simulink model "valida_angulo"  (R2023a)
settings: Solver=VariableStepAuto  StartTime=0.0  StopTime=10  RelTol=1e-3
values from neighbouring files (symbols this model uses):
  B = 0.3441    [datos_planta.m]
  J = 0.0112    [datos_planta.m]
  Jv = 13576.379e-12    (= 1.3576379e-08)    [datos_planta.m]
  Ka = 0.2335    [datos_planta.m]
  Km = 0.147    [datos_planta.m]
  L = 0.52    [datos_planta.m]
  R = 1.6    [datos_planta.m]
  Tm = 0.41    [datos_planta.m]
settings Model: Creator=hiago.sodre  LastModifiedBy=hiago.sodre

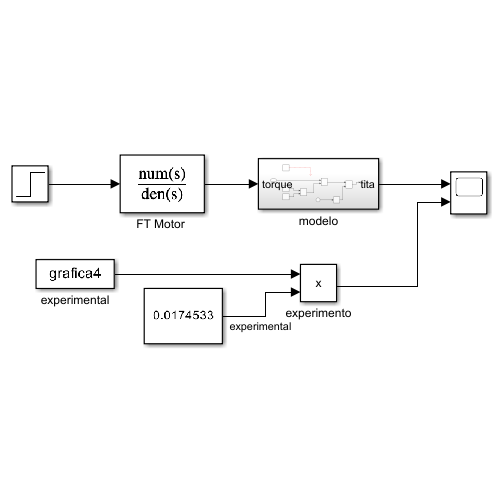
[thumbnail: Simulink's stored preview of the top-level diagram]
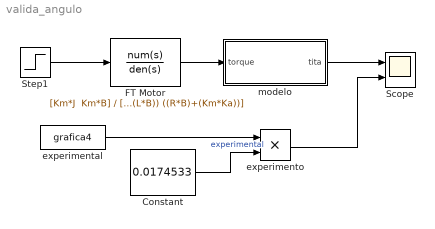
== system valida_angulo ==
  Constant : Constant  Value=0.0174533
  "FT Motor " : TransferFcn  Numerator="[Km*J  Km*B]"  Denominator=[L*J ((R*J)+(L*B)) ((R*B)+(Km*Ka))]
  Scope : Scope  NumInputPorts=2
  Step1 : Step  Time=0  After=5  SampleTime=0
  experimental : FromWorkspace  VariableName=grafica4
  experimento : Product  Inputs=**
  modelo : Subsystem
  wires:
  experimental/1 -> experimento/1
  Constant/1 -> experimento/2  "experimental"
  "FT Motor "/1 -> modelo/1(torque)
  Step1/1 -> "FT Motor "/1
  modelo/1(tita) -> Scope/1
  experimento/1 -> Scope/2

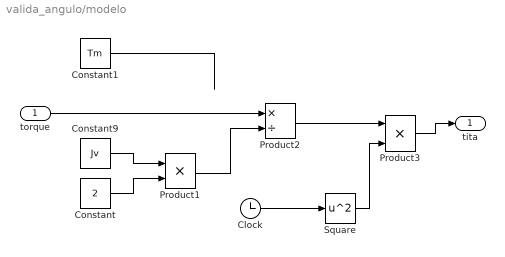
== system valida_angulo/modelo ==
  torque : Inport
  Clock : Clock
  Constant : Constant  Value=2
  Constant1 : Constant  Value=Tm
  Constant9 : Constant  Value=Jv
  Product1 : Product  Inputs=**
  Product2 : Product  Inputs=*/
  Product3 : Product  Inputs=**
  Square : Math  Operator=square
  tita : Outport
  wires:
  Constant9/1 -> Product1/1
  Constant/1 -> Product1/2
  Product1/1 -> Product2/2
  Constant1/1 -> ?
  torque/1 -> Product2/1
  Clock/1 -> Square/1
  Product2/1 -> Product3/1
  Square/1 -> Product3/2
  Product3/1 -> tita/1
